simulink model "levantamento"  (R2012b)
settings: Solver=ode45  StartTime=0.0  StopTime=1  RelTol=1e-3
undefined symbols (not defined in the file): fcem_a, fcem_b, fcem_c
libraries: simulink x7, BLDC x2, Tools x1
settings Model: Creator=h3now  LastModifiedBy=h3now

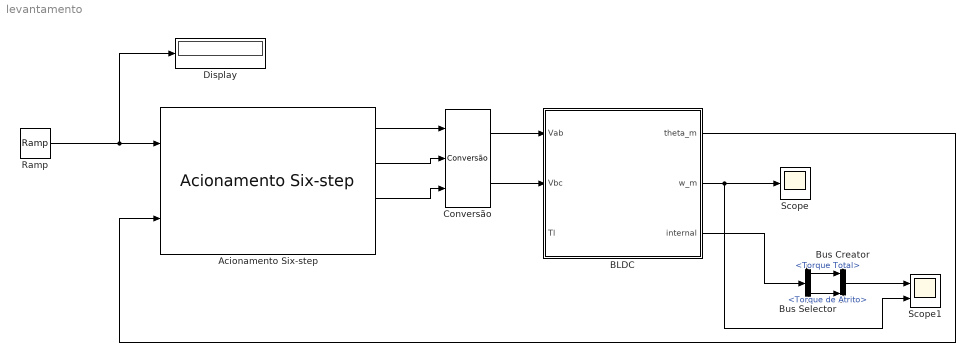
== system levantamento ==
  Acionamento Six-step : BLDC/Acionamento Six-step  P=8
  BLDC : Subsystem  mask(Simulador de um motor BLDC){J=1.39e-6, R=10.1/2, L=2.04/2000, P=8, Kt=15.7e-3/1.19, Ke=15.7e-3/1.19, Kd=0, F_stick=0.001, F_slip=0, default_fcem=on, fcem_a=fcem_a, fcem_b=fcem_b, fcem_c=fcem_c}
      mask prompts: J "Inércia do sistema motor+carga [Kg.m^2]"; R "Resistência por fase [Ohm]"; L "Indutância por fase (descontado o valor da indutância mútua, se for significativo) [Henry]"; P "Número de pólos"; Kt "Constante de torque [Nm/A]"; Ke "Constante de força eletromotriz [V.s] (numericamente igual à constante de torque se utilizar SI)"; Kd "Constante de atrito viscoso"; F_stick "Força máxima de atrito estático"; F_slip "Força de atrito dinâmico"; default_fcem "Utilizar back-emf trapezoidal?"; fcem_a "Lookup table da back-emf fase a"; fcem_b "Lookup table da back-emf fase b"; fcem_c "Lookup table da back-emf fase c"
      mask help:
      | Entradas
      | - Vab: Diferença de potencial entre a fase 'a' e a fase 'b' [V]
      | - Vbc: Diferença de potencial entre a fase 'b' e a fase 'c' [V]
      | - Tl: torque da carga [N.m]
      |
      | Saídas
      | - Theta_m: ângulo do rotor [rad]
      | - w_m: velocidade ângular do rotor [rad/s]
      | - internal: vetor de variáveis internas do simulador:
      |     - FCEM em cada fase [V] (3x1)
      |     - Corrente em cada fase [A] (3x1)
      |     - Torque produzido por cada fase [N.m] (3x1)
      |     - Torque total [N.m] (1x1)
      |     - Torque de atrito [N.m] (1x1)
      mask init:
      | % Se o usuário escolheu utilizar a back-emf padrão, inicializa as variáveis
      | % da lookuptables com valores zerados para não dar erro.
      | if default_fcem == 1
      |     fcem_a = [0,0;1,0];
      |     fcem_b = [0,0;1,0];
      |     fcem_c = [0,0;1,0];
      |     
      | % Se o usuário escolheu especificar qual será a forma da back-emf, checa se
      | % as lookup tables que ele inseriu fazem sentido.
      | else
      |     % Checa se a primeira coluna começa em 0.
      |     if fcem_a(1,1) ~= 0 ||fcem_b(1,1) ~= 0 || fcem_c(1,1) ~= 0
      |         error('A primeira coluna das lookup tables que definem o formato da back-emf devem começar em zero!');
      |     end
      |     % Checa se a primeira coluna termina em 360.
      |     if fcem_a(size(fcem_a,1),1) ~= 360 || fcem_b(size(fcem_b,1),1) ~= 360 || fcem_c(size(fcem_c,1),1) ~= 360
      |         error('A primeira coluna das lookup tables que definem o formato da back-emf deve terminar em 360!');
      |     end
      | end
      mask TypeOptions F_stick: Dinâmica mecânica /Atrito de coulomb/F_stick
      mask TypeOptions F_slip: Dinâmica mecânica /Atrito de coulomb/F_slip
      mask Callback default_fcem:
      | maskStr = get_param(gcb,'MaskValues');
      | 
      | if strcmp(maskStr{10},'on')
      |     set_param(gcb,'MaskVisibilities',{'on';'on';'on';'on';'on';'on';'on';'on';'on';'on';'off';'off';'off'});
      | else
      |     set_param(gcb,'MaskVisibilities',{'on';'on';'on';'on';'on';'on';'on';'on';'on';'on';'on';'on';'on'});
      | end
  Bus Creator : BusCreator  Inputs=2
  Bus Selector : BusSelector  OutputSignals=Torque Total,Torque de Atrito
  Conversão : BLDC/Conversão
  Display : Display
  Ramp : simulink/Sources/Ramp  slope=1  start=0  X0=0
  Scope : Scope
  Scope1 : Scope  NumInputPorts=2
      settings: ShowLegends=on  YMin=-5~-1  YMax=5~40
  wires:
  Conversão/1 -> BLDC/1(Vab)
  Conversão/2 -> BLDC/2(Vbc)
  Acionamento Six-step/1 -> Conversão/1
  Acionamento Six-step/2 -> Conversão/2
  Acionamento Six-step/3 -> Conversão/3
  BLDC/2(w_m) -> Scope/1, Scope1/2
  Ramp/1 -> Display/1, Acionamento Six-step/1
  BLDC/1(theta_m) -> Acionamento Six-step/2
  BLDC/3(internal) -> Bus Selector/1
  Bus Selector/1 -> Bus Creator/1  "<Torque Total>"
  Bus Selector/2 -> Bus Creator/2  "<Torque de Atrito>"
  Bus Creator/1 -> Scope1/1

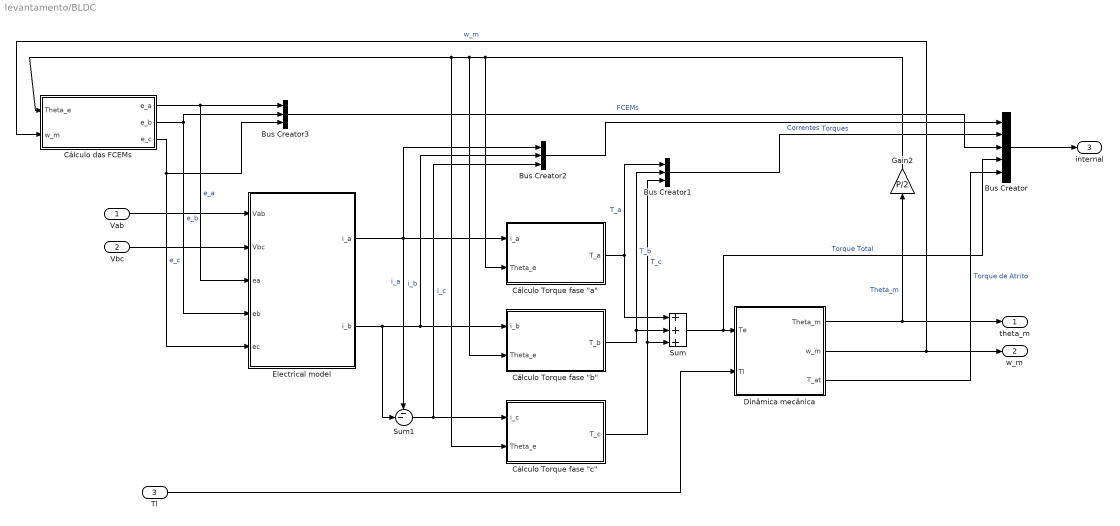
== system levantamento/BLDC ==
  Vab : Inport
  Vbc : Inport  Port=2
  Tl : Inport  Port=3
  Bus Creator : BusCreator  Inputs=5
  Bus Creator1 : BusCreator  Inputs=3
  Bus Creator2 : BusCreator  Inputs=3
  Bus Creator3 : BusCreator  Inputs=3
  "Cálculo Torque fase \"a\"" : Subsystem
  "Cálculo Torque fase \"b\"" : Subsystem
  "Cálculo Torque fase \"c\"" : Subsystem
  Cálculo das FCEMs : Subsystem
  "Dinâmica mecânica " : Subsystem
  Electrical model : Subsystem
  Gain2 : Gain  Gain=P/2
  Sum : Sum  Inputs=+++
  Sum1 : Sum  Inputs=--|
  theta_m : Outport
  w_m : Outport  Port=2
  internal : Outport  Port=3
  wires:
  Gain2/1 -> "Cálculo Torque fase \"b\""/2(Theta_e), Cálculo das FCEMs/1(Theta_e), "Cálculo Torque fase \"c\""/2(Theta_e), "Cálculo Torque fase \"a\""/2(Theta_e)
  Tl/1 -> "Dinâmica mecânica "/2(Tl)
  "Dinâmica mecânica "/2(w_m) -> Cálculo das FCEMs/2(w_m), w_m/1  "w_m"
  "Dinâmica mecânica "/1(Theta_m) -> Gain2/1, theta_m/1  "Theta_m"
  Sum/1 -> Bus Creator/4, "Dinâmica mecânica "/1(Te)  "Torque Total"
  "Cálculo Torque fase \"c\""/1(T_c) -> Bus Creator1/3, Sum/3  "T_c"
  "Cálculo Torque fase \"b\""/1(T_b) -> Bus Creator1/2, Sum/2  "T_b"
  "Cálculo Torque fase \"a\""/1(T_a) -> Bus Creator1/1, Sum/1  "T_a"
  Sum1/1 -> "Cálculo Torque fase \"c\""/1(i_c), Bus Creator2/3  "i_c"
  Electrical model/2(i_b) -> "Cálculo Torque fase \"b\""/1(i_b), Bus Creator2/2, Sum1/2  "i_b"
  Electrical model/1(i_a) -> "Cálculo Torque fase \"a\""/1(i_a), Bus Creator2/1, Sum1/1  "i_a"
  Vbc/1 -> Electrical model/2(Vbc)
  Cálculo das FCEMs/3(e_c) -> Electrical model/5(ec), Bus Creator3/3  "e_c"
  Cálculo das FCEMs/2(e_b) -> Electrical model/4(eb), Bus Creator3/2  "e_b"
  Cálculo das FCEMs/1(e_a) -> Electrical model/3(ea), Bus Creator3/1  "e_a"
  Bus Creator/1 -> internal/1
  Bus Creator3/1 -> Bus Creator/3  "FCEMs"
  Bus Creator2/1 -> Bus Creator/1  "Correntes"
  Bus Creator1/1 -> Bus Creator/2  "Torques"
  Vab/1 -> Electrical model/1(Vab)
  "Dinâmica mecânica "/3(T_at) -> Bus Creator/5  "Torque de Atrito"

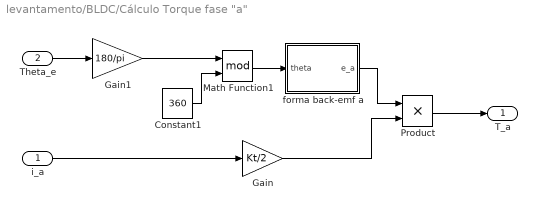
== system levantamento/BLDC/Cálculo Torque fase "a" ==
  i_a : Inport
  Theta_e : Inport  Port=2
  Constant1 : Constant  Value=360
  Gain : Gain  Gain=Kt/2
  Gain1 : Gain  Gain=180/pi
  Math Function1 : Math  Operator=mod  SaturateOnIntegerOverflow=on
  Product : Product  RndMeth=Zero
  forma back-emf a : Subsystem
  T_a : Outport
  wires:
  Constant1/1 -> Math Function1/2
  Gain1/1 -> Math Function1/1
  Product/1 -> T_a/1
  forma back-emf a/1(e_a) -> Product/1
  Theta_e/1 -> Gain1/1
  Math Function1/1 -> forma back-emf a/1(theta)
  Gain/1 -> Product/2
  i_a/1 -> Gain/1

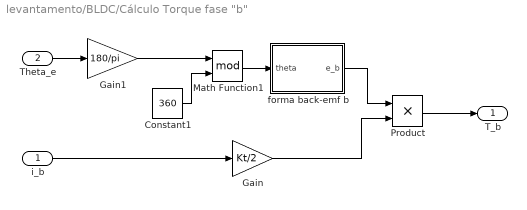
== system levantamento/BLDC/Cálculo Torque fase "b" ==
  i_b : Inport
  Theta_e : Inport  Port=2
  Constant1 : Constant  Value=360
  Gain : Gain  Gain=Kt/2
  Gain1 : Gain  Gain=180/pi
  Math Function1 : Math  Operator=mod  SaturateOnIntegerOverflow=on
  Product : Product  RndMeth=Zero
  forma back-emf b : Subsystem
  T_b : Outport
  wires:
  Constant1/1 -> Math Function1/2
  Gain1/1 -> Math Function1/1
  i_b/1 -> Gain/1
  Gain/1 -> Product/2
  Math Function1/1 -> forma back-emf b/1(theta)
  Theta_e/1 -> Gain1/1
  forma back-emf b/1(e_b) -> Product/1
  Product/1 -> T_b/1

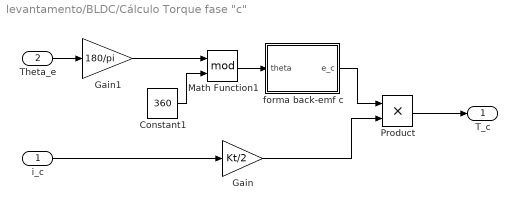
== system levantamento/BLDC/Cálculo Torque fase "c" ==
  i_c : Inport
  Theta_e : Inport  Port=2
  Constant1 : Constant  Value=360
  Gain : Gain  Gain=Kt/2
  Gain1 : Gain  Gain=180/pi
  Math Function1 : Math  Operator=mod  SaturateOnIntegerOverflow=on
  Product : Product  RndMeth=Zero
  forma back-emf c : Subsystem
  T_c : Outport
  wires:
  Constant1/1 -> Math Function1/2
  Gain1/1 -> Math Function1/1
  Product/1 -> T_c/1
  forma back-emf c/1(e_c) -> Product/1
  Theta_e/1 -> Gain1/1
  Math Function1/1 -> forma back-emf c/1(theta)
  Gain/1 -> Product/2
  i_c/1 -> Gain/1

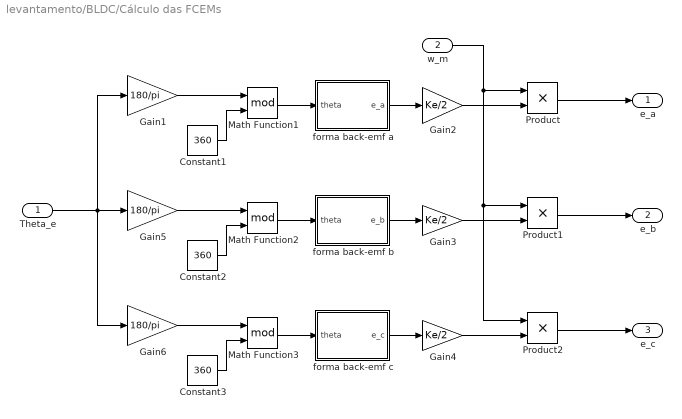
== system levantamento/BLDC/Cálculo das FCEMs ==
  Theta_e : Inport
  w_m : Inport  Port=2
  Constant1 : Constant  Value=360
  Constant2 : Constant  Value=360
  Constant3 : Constant  Value=360
  Gain1 : Gain  Gain=180/pi
  Gain2 : Gain  Gain=Ke/2
  Gain3 : Gain  Gain=Ke/2
  Gain4 : Gain  Gain=Ke/2
  Gain5 : Gain  Gain=180/pi
  Gain6 : Gain  Gain=180/pi
  Math Function1 : Math  Operator=mod  SaturateOnIntegerOverflow=on
  Math Function2 : Math  Operator=mod  SaturateOnIntegerOverflow=on
  Math Function3 : Math  Operator=mod  SaturateOnIntegerOverflow=on
  Product : Product  RndMeth=Zero
  Product1 : Product  RndMeth=Zero
  Product2 : Product  RndMeth=Zero
  forma back-emf a : Subsystem
  forma back-emf b : Subsystem
  forma back-emf c : Subsystem
  e_a : Outport
  e_b : Outport  Port=2
  e_c : Outport  Port=3
  wires:
  Constant3/1 -> Math Function3/2
  Constant2/1 -> Math Function2/2
  Constant1/1 -> Math Function1/2
  Product/1 -> e_a/1
  Product1/1 -> e_b/1
  Theta_e/1 -> Gain5/1, Gain1/1, Gain6/1
  Product2/1 -> e_c/1
  Gain2/1 -> Product/2
  w_m/1 -> Product/1, Product1/1, Product2/1
  Gain3/1 -> Product1/2
  Gain4/1 -> Product2/2
  Gain1/1 -> Math Function1/1
  Gain5/1 -> Math Function2/1
  Gain6/1 -> Math Function3/1
  Math Function1/1 -> forma back-emf a/1(theta)
  forma back-emf a/1(e_a) -> Gain2/1
  Math Function2/1 -> forma back-emf b/1(theta)
  forma back-emf b/1(e_b) -> Gain3/1
  Math Function3/1 -> forma back-emf c/1(theta)
  forma back-emf c/1(e_c) -> Gain4/1

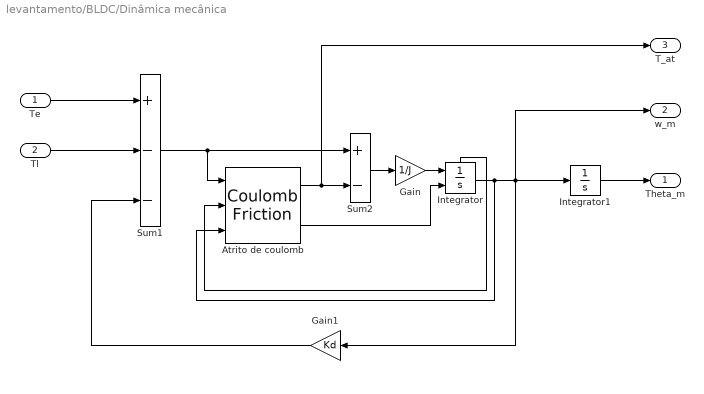
== system levantamento/BLDC/Dinâmica mecânica  ==
  Te : Inport
  Tl : Inport  Port=2
  Atrito de coulomb : Tools/Coulomb Friction  F_stick=F_stick  F_slip=F_slip
  Gain : Gain  Gain=1/J
  Gain1 : Gain  Gain=Kd
  Integrator : Integrator  ExternalReset=rising  ShowStatePort=on
  Integrator1 : Integrator
  Sum1 : Sum  Inputs=+--
  Sum2 : Sum  Inputs=+-
  Theta_m : Outport
  w_m : Outport  Port=2
  T_at : Outport  Port=3
  wires:
  Integrator1/1 -> Theta_m/1
  Tl/1 -> Sum1/2
  Gain1/1 -> Sum1/3
  Te/1 -> Sum1/1
  Integrator/1 -> Atrito de coulomb/3, w_m/1, Integrator1/1, Gain1/1
  Gain/1 -> Integrator/1
  Sum2/1 -> Gain/1
  Sum1/1 -> Sum2/1, Atrito de coulomb/1
  Atrito de coulomb/1 -> T_at/1, Sum2/2
  Atrito de coulomb/2 -> Integrator/2
  Integrator/State -> Atrito de coulomb/2

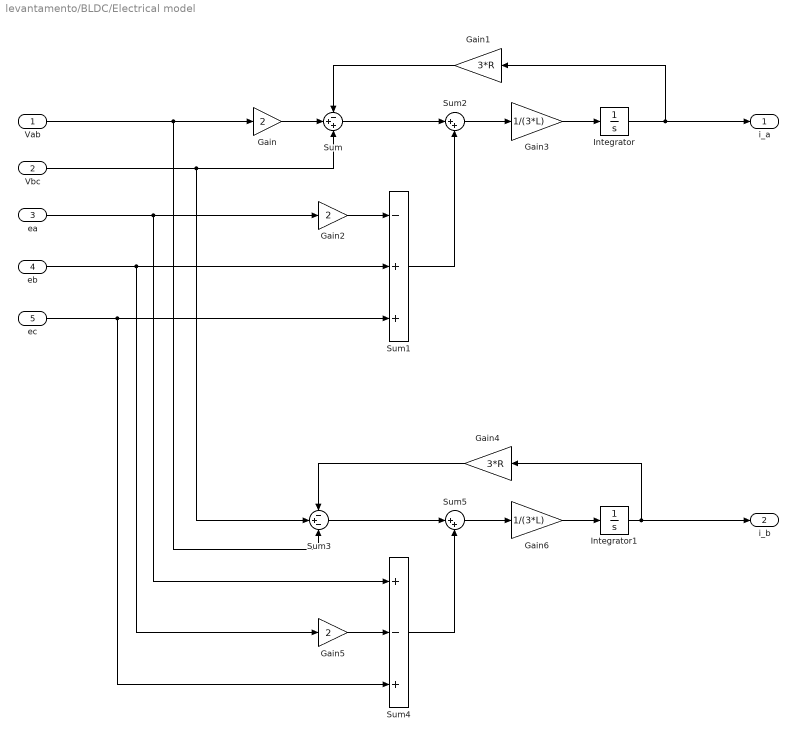
== system levantamento/BLDC/Electrical model ==
  Vab : Inport
  Vbc : Inport  Port=2
  ea : Inport  Port=3
  eb : Inport  Port=4
  ec : Inport  Port=5
  Gain : Gain  Gain=2
  Gain1 : Gain  Gain=3*R
  Gain2 : Gain  Gain=2
  Gain3 : Gain  Gain=1/(3*L)
  Gain4 : Gain  Gain=3*R
  Gain5 : Gain  Gain=2
  Gain6 : Gain  Gain=1/(3*L)
  Integrator : Integrator
  Integrator1 : Integrator
  Sum : Sum  Inputs=-++
  Sum1 : Sum  Inputs=-++
  Sum2 : Sum  Inputs=|++
  Sum3 : Sum  Inputs=-+-
  Sum4 : Sum  Inputs=+-+
  Sum5 : Sum  Inputs=|++
  i_a : Outport
  i_b : Outport  Port=2
  wires:
  Gain6/1 -> Integrator1/1
  Gain5/1 -> Sum4/2
  Sum3/1 -> Sum5/1
  Sum4/1 -> Sum5/2
  Sum5/1 -> Gain6/1
  Gain2/1 -> Sum1/1
  ea/1 -> Sum4/1, Gain2/1
  Gain1/1 -> Sum/1
  Integrator/1 -> i_a/1, Gain1/1
  Gain/1 -> Sum/2
  Vab/1 -> Sum3/3, Gain/1
  Sum2/1 -> Gain3/1
  Gain3/1 -> Integrator/1
  ec/1 -> Sum4/3, Sum1/3
  eb/1 -> Gain5/1, Sum1/2
  Sum1/1 -> Sum2/2
  Sum/1 -> Sum2/1
  Vbc/1 -> Sum3/2, Sum/3
  Gain4/1 -> Sum3/1
  Integrator1/1 -> i_b/1, Gain4/1

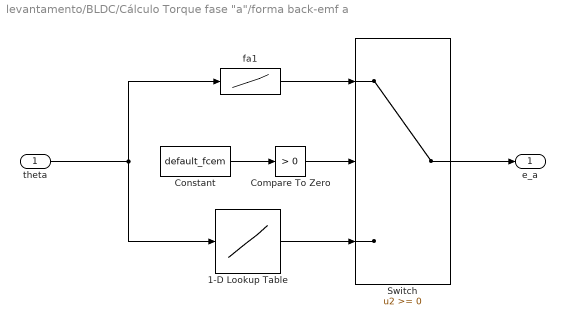
== system levantamento/BLDC/Cálculo Torque fase "a"/forma back-emf a ==
  theta : Inport
  1-D Lookup Table : Lookup_n-D  NumberOfTableDimensions=1  BreakpointsForDimension1=fcem_a(:,1)  Table=fcem_a(:,2)  RndMeth=Simplest  InputSameDT=on
  Compare To Zero : simulink/Logic and Bit Operations/Compare To Zero  relop=>  OutDataTypeStr=boolean
  Constant : Constant  Value=default_fcem
  Switch : Switch
  fa1 : Lookup  InputValues=[0 30 60 90 120 150 180 210 240 270 300 330 360]  Table=[ 1 1 1 0 -1 -1 -1 -1 -1 0 1 1 1]
  e_a : Outport
  wires:
  theta/1 -> 1-D Lookup Table/1, fa1/1
  Switch/1 -> e_a/1
  fa1/1 -> Switch/1
  1-D Lookup Table/1 -> Switch/3
  Compare To Zero/1 -> Switch/2
  Constant/1 -> Compare To Zero/1

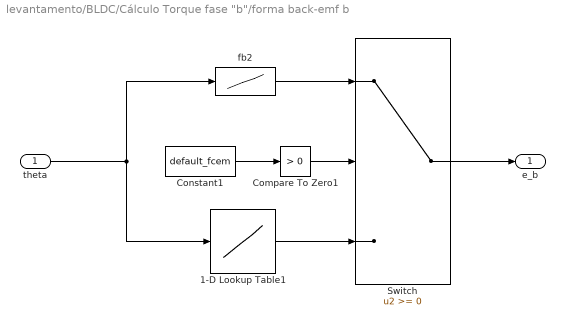
== system levantamento/BLDC/Cálculo Torque fase "b"/forma back-emf b ==
  theta : Inport
  1-D Lookup Table1 : Lookup_n-D  NumberOfTableDimensions=1  BreakpointsForDimension1=fcem_b(:,1)  Table=fcem_b(:,2)  RndMeth=Simplest  InputSameDT=on
  Compare To Zero1 : simulink/Logic and Bit Operations/Compare To Zero  relop=>  OutDataTypeStr=boolean
  Constant1 : Constant  Value=default_fcem
  Switch : Switch
  fb2 : Lookup  InputValues=[0 30 60 90 120 150 180 210 240 270 300 330 360]  Table=[-1 0 1 1 1 1 1 0 -1 -1 -1 -1 -1]
  e_b : Outport
  wires:
  1-D Lookup Table1/1 -> Switch/3
  theta/1 -> 1-D Lookup Table1/1, fb2/1
  Compare To Zero1/1 -> Switch/2
  Constant1/1 -> Compare To Zero1/1
  Switch/1 -> e_b/1
  fb2/1 -> Switch/1

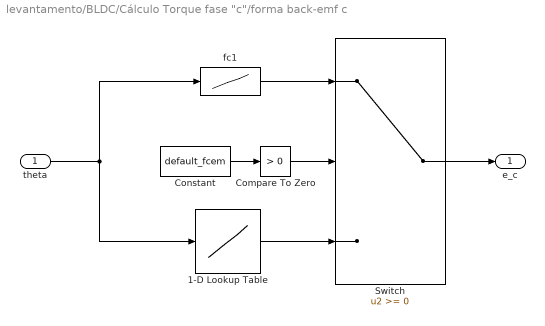
== system levantamento/BLDC/Cálculo Torque fase "c"/forma back-emf c ==
  theta : Inport
  1-D Lookup Table : Lookup_n-D  NumberOfTableDimensions=1  BreakpointsForDimension1=fcem_c(:,1)  Table=fcem_c(:,2)  RndMeth=Simplest  InputSameDT=on
  Compare To Zero : simulink/Logic and Bit Operations/Compare To Zero  relop=>  OutDataTypeStr=boolean
  Constant : Constant  Value=default_fcem
  Switch : Switch
  fc1 : Lookup  InputValues=[0 30 60 90 120 150 180 210 240 270 300 330 360]  Table=[-1 -1 -1 -1 -1 0 1 1 1 1 1 0 -1]
  e_c : Outport
  wires:
  1-D Lookup Table/1 -> Switch/3
  theta/1 -> 1-D Lookup Table/1, fc1/1
  Compare To Zero/1 -> Switch/2
  Constant/1 -> Compare To Zero/1
  Switch/1 -> e_c/1
  fc1/1 -> Switch/1

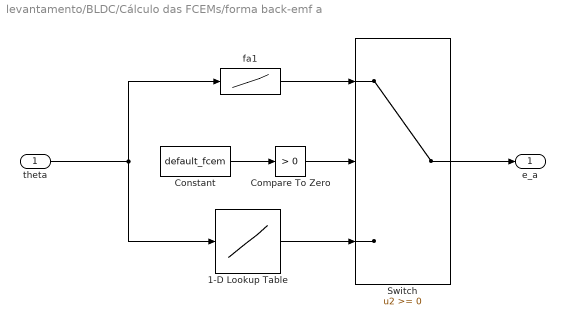
== system levantamento/BLDC/Cálculo das FCEMs/forma back-emf a ==
  theta : Inport
  1-D Lookup Table : Lookup_n-D  NumberOfTableDimensions=1  BreakpointsForDimension1=fcem_a(:,1)  Table=fcem_a(:,2)  RndMeth=Simplest  InputSameDT=on
  Compare To Zero : simulink/Logic and Bit Operations/Compare To Zero  relop=>  OutDataTypeStr=boolean
  Constant : Constant  Value=default_fcem
  Switch : Switch
  fa1 : Lookup  InputValues=[0 30 60 90 120 150 180 210 240 270 300 330 360]  Table=[ 1 1 1 0 -1 -1 -1 -1 -1 0 1 1 1]
  e_a : Outport
  wires:
  theta/1 -> 1-D Lookup Table/1, fa1/1
  Switch/1 -> e_a/1
  fa1/1 -> Switch/1
  1-D Lookup Table/1 -> Switch/3
  Compare To Zero/1 -> Switch/2
  Constant/1 -> Compare To Zero/1

== system levantamento/BLDC/Cálculo das FCEMs/forma back-emf b ==
  theta : Inport
  1-D Lookup Table1 : Lookup_n-D  NumberOfTableDimensions=1  BreakpointsForDimension1=fcem_b(:,1)  Table=fcem_b(:,2)  RndMeth=Simplest  InputSameDT=on
  Compare To Zero1 : simulink/Logic and Bit Operations/Compare To Zero  relop=>  OutDataTypeStr=boolean
  Constant1 : Constant  Value=default_fcem
  Switch : Switch
  fb2 : Lookup  InputValues=[0 30 60 90 120 150 180 210 240 270 300 330 360]  Table=[-1 0 1 1 1 1 1 0 -1 -1 -1 -1 -1]
  e_b : Outport
  wires:
  1-D Lookup Table1/1 -> Switch/3
  theta/1 -> 1-D Lookup Table1/1, fb2/1
  Compare To Zero1/1 -> Switch/2
  Constant1/1 -> Compare To Zero1/1
  Switch/1 -> e_b/1
  fb2/1 -> Switch/1

== system levantamento/BLDC/Cálculo das FCEMs/forma back-emf c ==
  theta : Inport
  1-D Lookup Table : Lookup_n-D  NumberOfTableDimensions=1  BreakpointsForDimension1=fcem_c(:,1)  Table=fcem_c(:,2)  RndMeth=Simplest  InputSameDT=on
  Compare To Zero : simulink/Logic and Bit Operations/Compare To Zero  relop=>  OutDataTypeStr=boolean
  Constant : Constant  Value=default_fcem
  Switch : Switch
  fc1 : Lookup  InputValues=[0 30 60 90 120 150 180 210 240 270 300 330 360]  Table=[-1 -1 -1 -1 -1 0 1 1 1 1 1 0 -1]
  e_c : Outport
  wires:
  1-D Lookup Table/1 -> Switch/3
  theta/1 -> 1-D Lookup Table/1, fc1/1
  Compare To Zero/1 -> Switch/2
  Constant/1 -> Compare To Zero/1
  Switch/1 -> e_c/1
  fc1/1 -> Switch/1
